simulink model "ventilator"  (R2020a)
settings: Solver=VariableStepAuto  StartTime=0.0  StopTime=20  FixedStep=0.001  MaxStep=0.01  RelTol=1e-3  AbsTol=1e-3
PreLoadFcn:
  | addpath('../controller');
PostLoadFcn:
  | load('params');
InitFcn:
  | load('params');
  | 
  | Transport_Delay = 0.001; % s
  | 
  | P_supply = 4; % bar
  | P_regulator = 0.75; % bar
  | FiO2 = 0.6;
  | 
  | Sensors_Ts = 0.01; % s
  | Zephyr_FS = 50; % SLPM
  | HSC_LP_FS = 160; % mbar
  | HSC_HP_FS = 10000; % mbar
  | 
  | HEPA_ratio = 5 / 20; % mbar / L/min
  | 
  | T_room = 20; % degC
  | RH_room = 0.1;
  | T_humidifier = 40; % degC
  | T_body = 37; % degC
  | 
  | L_tube = 1; % m
  | D_tube = 0.022; % m
  | L_trachea = 0.15; % m
  | D_trachea = 0.015; % m
  | 
  | Chamber_volume = 0.2; % L
  | FRC = 2; % L
  | 
  | cmH2O_to_Pa = 98.0665;
undefined symbols (not defined in the file or in its folder): tc, zephyr
libraries: fl_lib x158, nesl_utility x18, simulink x2
(part 1 of 3)
CloseFcn:
  | clear Transport_Delay
  | clear P_supply P_regulator FiO2
  | clear Sensors_Ts Zephyr_FS HSC_LP_FS HSC_HP_FS
  | clear HEPA_ratio
  | clear T_room RH_room T_humidifier T_body
  | clear L_tube D_tube L_trachea D_trachea
  | clear Chamber_volume FRC
  | clear cmH2O_to_Pa
  | 
  | rmpath('../controller');
Description:
  | Medical Ventilator IIT-Ferrari-Camozzi
settings Model: Creator=MathWorks  LastModifiedBy=upattacini
settings SolverCC: AutoScaleAbsTol=off  MaxConsecutiveMinStep=10  ZeroCrossAlgorithm=Adaptive  AlgebraicLoopSolver=LineSearch
settings DataIOCC: SaveOutput=off  SignalLogging=off  DSMLogging=off  SaveTime=off  ReturnWorkspaceOutputs=off
settings DebuggingCC: IgnoredZcDiagnostic=none  PregeneratedLibrarySubsystemCodeDiagnostic=none  ArithmeticOperatorsInVariantConditions=warning
settings SFSimCC: SimUseLocalCustomCode=off  CustomCodeUndefinedFunction=UseInterfaceOnly
settings RTWCC: RTWUseLocalCustomCode=off
settings SimscapeCC: SimscapeLogName=simlog_ventilator  SimscapeLogDataHistory=10000

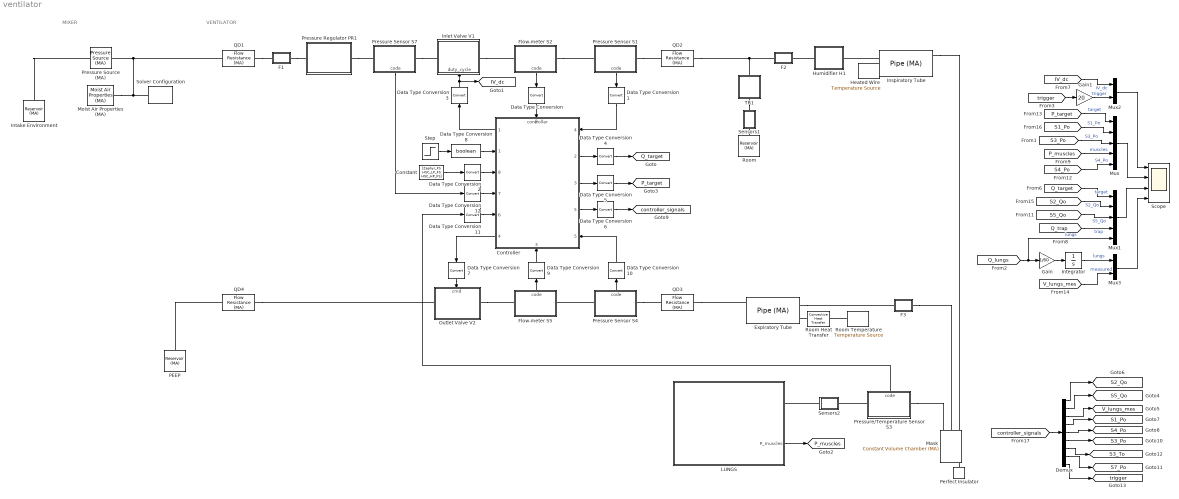
== system ventilator ==
  note: MIXER
  note: VENTILATOR
  Constant : Constant  Value=[Zephyr_FS HSC_LP_FS HSC_HP_FS]
  Controller : ModelReference  ModelNameDialog=controller.slx  SimulationMode=Normal  ModelReferenceVersion=1.393
      settings: PortSchema="{\"entries\":[{\"content\":{\"sides\":[{\"content\":{\"connectorIds\":[\"Out1\",\"In1\",\"In8\",\"In7\",\"In6\",\"Out4\"]},\"type\":\"ConnectorPlacement.EquallySpacedRectSide\",\"uuid\":\"dfd9e8e3-11ff-4499-8101-aea092fe61dc\"},{\"content\":{\"connectorIds\":[\"In4\",\"Out2\",\"Out3\",\"Out5\",\"In5\"],\"side\":\"RIGHT\"},\"type\":\"ConnectorPlacement.EquallySpacedRectSide\",\"uuid\":\"77ce251b-d568-4b78-9724-05f123a60627\"},{\"content\":{\"connectorIds\":[\"In2\"],\"side\":\"TOP\"},\"type\":\"ConnectorPlacement.EquallySpacedRectSide\",\"uuid\":\"86366d86-38ff-4f13-9006-68bedaa415c8\"},{\"content\":{\"connectorIds\":[\"In3\"],\"side\":\"BOTTOM\"},\"type\":\"ConnectorPlacement.EquallySpacedRectSide\",\"uuid\":\"bf42dafa-2a5f-47c5-a086-0e16cdc85087\"}]},\"type\":\"ConnectorPlacement.EquallySpacedConnector\",\"uuid\":\"7cf5e0c6-4e76-497f-b162-c8492159840b\"}],\"packageUris\":[\"http://schema.mathworks.com/mf0/Connector/19700101\"],\"version\":\"1.0\"}"
  Data Type Conversion{,1..7,9..12} (12 alike) : DataTypeConversion
  Data Type Conversion8 : DataTypeConversion  OutDataTypeStr=boolean
  Demux : Demux  Outputs=9
  Expiratory Tube : fl_lib/Moist Air/Elements/Pipe (MA)  length=L_tube m  area=pi*D_tube^2/4 m^2  Dh=D_tube m  length_add=0.1 m  roughness=15e-6 m  Re_lam=2000  Re_tur=4000  shape_factor=64  Nu_lam=3.66  RH_ws=1  time_constant=1e-3 s  moisture_trace_gas_source=foundation.enum.moisture_trace_gas_source.none  moisture_source_spec=foundation.enum.moisture_source_spec.vapor  moisture_mass_flow=0 kg/s  moisture_temperature_spec=foundation.enum.temperature_spec.atmospheric  moisture_temperature=293.15 K  trace_gas_mass_flow=0 kg/s  trace_gas_temperature_spec=foundation.enum.temperature_spec.atmospheric  trace_gas_temperature=293.15 K  p_I_specify=off  p_I_priority=High  p_I=0.101325 MPa  p_I_nominal_specify=off  p_I_nominal_unit=MPa  p_I_nominal_value=1  T_I_specify=on  T_I_priority=High  T_I=T_room degC  T_I_nominal_specify=off  T_I_nominal_unit=K  T_I_nominal_value=1  RH_I_specify=on  RH_I_priority=High  RH_I=RH_room  RH_I_nominal_specify=off  RH_I_nominal_unit=1  RH_I_nominal_value=1  x_w_I_specify=off  x_w_I_priority=None  x_w_I=0  x_w_I_nominal_specify=off  x_w_I_nominal_unit=1  x_w_I_nominal_value=1  y_w_I_specify=off  y_w_I_priority=None  y_w_I=0  y_w_I_nominal_specify=off  y_w_I_nominal_unit=1  y_w_I_nominal_value=1  HR_I_specify=off  HR_I_priority=None  HR_I=0  HR_I_nominal_specify=off  HR_I_nominal_unit=1  HR_I_nominal_value=1  x_g_I_specify=off  x_g_I_priority=High  x_g_I=0  x_g_I_nominal_specify=off  x_g_I_nominal_unit=1  x_g_I_nominal_value=1  y_g_I_specify=off  y_g_I_priority=None  y_g_I=0  y_g_I_nominal_specify=off  y_g_I_nominal_unit=1  y_g_I_nominal_value=1
      settings: SourceProductBaseCode=MT,SS
  F1 : Subsystem  mask(Filter){ratio=HEPA_ratio}
      mask prompts: ratio "Pressure Loss / Fow Ratio (mbar / L/m)"
      mask help: HEPA air filtering.
  F2 : Subsystem  mask(Filter){ratio=HEPA_ratio}
      mask prompts: ratio "Pressure Loss / Fow Ratio (mbar / L/m)"
      mask help: HEPA air filtering.
  F3 : Subsystem  mask(Filter){ratio=HEPA_ratio}
      mask prompts: ratio "Pressure Loss / Fow Ratio (mbar / L/m)"
      mask help: HEPA air filtering.
  Flow-meter S2 : Subsystem  mask(Zephyr Airflow){FS=Zephyr_FS, Ts=Sensors_Ts}
      mask prompts: FS "Full Scale (SLPM)"; Ts "Sample Time (s)"
      mask help: Flow-meter with given characteristics.
      settings: PortSchema="{\"entries\":[{\"content\":{\"sides\":[{\"content\":{\"connectorIds\":[\"LConn1\"]},\"type\":\"ConnectorPlacement.EquallySpacedRectSide\",\"uuid\":\"3eddd698-891c-467d-aa25-3b16d36954ee\"},{\"content\":{\"connectorIds\":[\"RConn1\"],\"side\":\"RIGHT\"},\"type\":\"ConnectorPlacement.EquallySpacedRectSide\",\"uuid\":\"03609a73-c50b-4e66-9a76-94e8c0ebe662\"},{\"content\":{\"connectorIds\":[],\"side\":\"TOP\"},\"type\":\"ConnectorPlacement.EquallySpacedRectSide\",\"uuid\":\"5e48618e-d044-446b-90d3-a440c85d800d\"},{\"content\":{\"connectorIds\":[\"Out1\"],\"side\":\"BOTTOM\"},\"type\":\"ConnectorPlacement.EquallySpacedRectSide\",\"uuid\":\"0cc54025-99cb-4d46-b4e7-784a240d207c\"}]},\"type\":\"ConnectorPlacement.EquallySpacedConnector\",\"uuid\":\"f0fac613-21b7-4ef5-8119-2acb00be7d29\"}],\"packageUris\":[\"http://schema.mathworks.com/mf0/Connector/19700101\"],\"version\":\"1.0\"}"
      mask Display: image('../assets/honeywell.png');
  Flow-meter S5 : Subsystem  mask(Zephyr Airflow){FS=Zephyr_FS, Ts=Sensors_Ts}
      mask prompts: FS "Full Scale (SLPM)"; Ts "Sample Time (s)"
      mask help: Flow-meter with given characteristics.
      settings: PortSchema="{\"entries\":[{\"content\":{\"sides\":[{\"content\":{\"connectorIds\":[\"LConn1\"]},\"type\":\"ConnectorPlacement.EquallySpacedRectSide\",\"uuid\":\"3eddd698-891c-467d-aa25-3b16d36954ee\"},{\"content\":{\"connectorIds\":[\"RConn1\"],\"side\":\"RIGHT\"},\"type\":\"ConnectorPlacement.EquallySpacedRectSide\",\"uuid\":\"03609a73-c50b-4e66-9a76-94e8c0ebe662\"},{\"content\":{\"connectorIds\":[],\"side\":\"TOP\"},\"type\":\"ConnectorPlacement.EquallySpacedRectSide\",\"uuid\":\"5e48618e-d044-446b-90d3-a440c85d800d\"},{\"content\":{\"connectorIds\":[\"Out1\"],\"side\":\"BOTTOM\"},\"type\":\"ConnectorPlacement.EquallySpacedRectSide\",\"uuid\":\"0cc54025-99cb-4d46-b4e7-784a240d207c\"}]},\"type\":\"ConnectorPlacement.EquallySpacedConnector\",\"uuid\":\"f0fac613-21b7-4ef5-8119-2acb00be7d29\"}],\"packageUris\":[\"http://schema.mathworks.com/mf0/Connector/19700101\"],\"version\":\"1.0\"}"
      mask Display: image('../assets/honeywell.png');
  Gain : Gain  Gain=1/60
  Gain1 : Gain  Gain=20
  Heated Wire : fl_lib/Thermal/Thermal Sources/Temperature Source  temperature=T_body degC
      settings: SourceProductBaseCode=MT,SS
  Humidifier H1 : Subsystem  Tag=PublishSubsystem  mask(Humidifier){T_water=T_humidifier, A_humidifier=0.025, V_humidifier=0.001}
      mask prompts: T_water "Water temperature (degC)"; A_humidifier "Water surface area (m^2)"; V_humidifier "Air volume (m^3)"
      mask help: This subsystem models an active passover humidifier to increase moisture in the inspiratory flow.
  Inlet Valve V1 : Subsystem  mask(Proportional Valve){valve_type=CP, ap_tau_em=0.01/4, ap_tau_flow=0.045/4, cp_tau=0.02/4, cp_dead_time=0.01}
      mask prompts: valve_type "Valve Type"; ap_tau_em "Electromechanical Time Constant (s)"; ap_tau_flow "Flow Rate Time Constant (s)"; cp_tau "Time Constant (s)"; cp_dead_time "Dead Time (s)"
      mask help:
      | The valve is characterized by diagrams relating duty cycle, flow rate, and pressure loss.
      | The input is the PWM duty cycle.
      mask init:
      | if valve_type == 1
      |     valve = evalin('base','ap');
      | else
      |     valve = evalin('base','cp');
      | end
      settings: PortSchema="{\"entries\":[{\"content\":{\"sides\":[{\"content\":{\"connectorIds\":[\"LConn1\"]},\"type\":\"ConnectorPlacement.EquallySpacedRectSide\",\"uuid\":\"0b0135b1-d7b1-428e-90f3-2a98bec52953\"},{\"content\":{\"connectorIds\":[\"RConn1\"],\"side\":\"RIGHT\"},\"type\":\"ConnectorPlacement.EquallySpacedRectSide\",\"uuid\":\"8225685a-6f4e-4f4e-a754-9e90146eeb84\"},{\"content\":{\"connectorIds\":[\"In1\"],\"side\":\"TOP\"},\"type\":\"ConnectorPlacement.EquallySpacedRectSide\",\"uuid\":\"19c5f21c-927f-4e6e-aef1-94ad3534e6af\"}]},\"type\":\"ConnectorPlacement.EquallySpacedConnector\",\"uuid\":\"ea880819-6bb4-4c70-964b-d5a8d420d61d\"}],\"packageUris\":[\"http://schema.mathworks.com/mf0/Connector/19700101\"],\"version\":\"1.0\"}"
      mask TypeOptions valve_type: AP | CP
      mask Callback valve_type:
      | numparams = Simulink.Mask.get(gcb).numParameters;
      | enable = cell(1, numparams);
      | enable(:) = {'on'};
      | 
      | mode = get_param(gcb, 'valve_type');
      | if strcmpi(mode, 'CP')
      |     enable(2:3) = {'off'};
      | else
      |     enable(4:5) = {'off'};
      | end
      | set_param(gcb, 'MaskEnables', enable);
      mask Display: image('../assets/camozzi.jpg');
  Inspiratory Tube : fl_lib/Moist Air/Elements/Pipe (MA)  length=L_tube m  area=pi*D_tube^2/4 m^2  Dh=D_tube m  length_add=0.1 m  roughness=15e-6 m  Re_lam=2000  Re_tur=4000  shape_factor=64  Nu_lam=3.66  RH_ws=1  time_constant=1e-3 s  moisture_trace_gas_source=foundation.enum.moisture_trace_gas_source.none  moisture_source_spec=foundation.enum.moisture_source_spec.vapor  moisture_mass_flow=0 kg/s  moisture_temperature_spec=foundation.enum.temperature_spec.atmospheric  moisture_temperature=293.15 K  trace_gas_mass_flow=0 kg/s  trace_gas_temperature_spec=foundation.enum.temperature_spec.atmospheric  trace_gas_temperature=293.15 K  p_I_specify=off  p_I_priority=High  p_I=0.101325 MPa  p_I_nominal_specify=off  p_I_nominal_unit=MPa  p_I_nominal_value=1  T_I_specify=on  T_I_priority=High  T_I=T_room degC  T_I_nominal_specify=off  T_I_nominal_unit=K  T_I_nominal_value=1  RH_I_specify=on  RH_I_priority=High  RH_I=RH_room  RH_I_nominal_specify=off  RH_I_nominal_unit=1  RH_I_nominal_value=1  x_w_I_specify=off  x_w_I_priority=None  x_w_I=0  x_w_I_nominal_specify=off  x_w_I_nominal_unit=1  x_w_I_nominal_value=1  y_w_I_specify=off  y_w_I_priority=None  y_w_I=0  y_w_I_nominal_specify=off  y_w_I_nominal_unit=1  y_w_I_nominal_value=1  HR_I_specify=off  HR_I_priority=None  HR_I=0  HR_I_nominal_specify=off  HR_I_nominal_unit=1  HR_I_nominal_value=1  x_g_I_specify=off  x_g_I_priority=High  x_g_I=0  x_g_I_nominal_specify=off  x_g_I_nominal_unit=1  x_g_I_nominal_value=1  y_g_I_specify=off  y_g_I_priority=None  y_g_I=0  y_g_I_nominal_specify=off  y_g_I_nominal_unit=1  y_g_I_nominal_value=1
      settings: SourceProductBaseCode=MT,SS
  Intake Environment : fl_lib/Moist Air/Elements/Reservoir (MA)  pressure_spec=foundation.enum.pressure_spec.atmospheric  reservoir_pressure=P_supply bar  temperature_spec=foundation.enum.temperature_spec.specified  reservoir_temperature=T_room degC  moisture_spec=foundation.enum.moisture_spec.relative_humidity  reservoir_RH=RH_room  reservoir_x_w=0.01  reservoir_y_w=0.01  reservoir_HR=0.01  trace_gas_spec=foundation.enum.trace_gas_spec.mole_fraction  reservoir_x_g=0  reservoir_y_g=FiO2  RH_ws=1  area_A=pi*D_tube^2/4 m^2
      settings: SourceProductBaseCode=MT,SS
  Integrator : Integrator
  LUNGS : Subsystem  mask(Lungs){lungs_type=Medium, muscles_enabled=off, p_muscles_mag=10, t_inhale=0.5, t_exhale=1, period=5, delay=1.1}
      mask prompts: lungs_type "Lungs Type"; muscles_enabled "Enable Muscles Pressure"; p_muscles_mag "Muscles pressure magnitude (cmH20)"; t_inhale "Inhalation duration (s)"; t_exhale "Exhalation duration (s)"; period "Period (s)"; delay "Delay (s)"
      mask help:
      | This subsystem accounts for the lungs dynamics resorting to a translational mechanical converter that is responsible for converting moist air in volume change.
      |
      | Because the interface cross-sectional area parameter is set to 1 m^2, therefore 1 m of measured displacement is equivalent to 1 m^3 of lungs volume and 1 N of measured force is equivalent to 1 Pa of pressure.
      mask init:
      | lungs_compliant = struct('Em',60,'E',2.6,'Rm',0.9,'R0',0.47,'Kv',-0.45,'Kf',0.01);
      | lungs_medium = struct('Em',60,'E',5.9,'Rm',0.4,'R0',0.3,'Kv',-0.35,'Kf',0.4);
      | lungs_stiff = struct('Em',60,'E',9.1,'Rm',0.85,'R0',0.1,'Kv',-0.6,'Kf',0.8);
      | 
      | if lungs_type == 1
      |     lungs = lungs_compliant;
      | elseif lungs_type == 2
      |     lungs = lungs_medium;
      | else
      |     lungs = lungs_stiff;
      | end
      settings: PortSchema="{\"entries\":[{\"content\":{\"sides\":[{\"content\":{\"connectorIds\":[]},\"type\":\"ConnectorPlacement.EquallySpacedRectSide\",\"uuid\":\"d76c9f72-7b8e-4684-b79a-2f479b0f4ef9\"},{\"content\":{\"connectorIds\":[\"RConn1\",\"Out1\"],\"side\":\"RIGHT\"},\"type\":\"ConnectorPlacement.EquallySpacedRectSide\",\"uuid\":\"9c49ecd1-09fc-45b8-94ed-4278a65fc871\"},{\"content\":{\"connectorIds\":[],\"side\":\"TOP\"},\"type\":\"ConnectorPlacement.EquallySpacedRectSide\",\"uuid\":\"c20a617e-bdd3-44e9-88c4-f17e0ef57963\"}]},\"type\":\"ConnectorPlacement.EquallySpacedConnector\",\"uuid\":\"46ba8907-2938-4721-a0f5-c6c7a7a60368\"}],\"packageUris\":[\"http://schema.mathworks.com/mf0/Connector/19700101\"],\"version\":\"1.0\"}"
      mask TypeOptions lungs_type: Compliant | Medium | Stiff
      mask Callback muscles_enabled:
      | numparams = Simulink.Mask.get(gcb).numParameters;
      | enable = cell(1, numparams);
      | enable(:) = {'on'};
      | h = Simulink.findBlocks(gcb, 'Name' , 'Muscles Pressure Waveform');
      | 
      | mode = get_param(gcb, 'muscles_enabled');
      | if strcmpi(mode, 'on')
      |     set_param(h, 'Commented', 'off');
      | else
      |     set_param(h, 'Commented', 'on');
      |     enable(3:end) = {'off'};
      | end
      | set_param(gcb, 'MaskEnables', enable);
      mask DialogControl Container1 Prompt: Parameters
      mask Display: image('../assets/lungs.png');
  Mask : fl_lib/Moist Air/Elements/Constant Volume Chamber (MA)  volume=Chamber_volume l  num_ports=foundation.enum.num_ports.three  area_A=pi*D_trachea^2/4 m^2  area_B=pi*D_tube^2/4 m^2  area_C=pi*D_tube^2/4 m^2  area_D=0.01 m^2  RH_ws=1  time_constant=1e-3 s  moisture_trace_gas_source=foundation.enum.moisture_trace_gas_source.none  moisture_source_spec=foundation.enum.moisture_source_spec.vapor  moisture_mass_flow=0 kg/s  moisture_temperature_spec=foundation.enum.temperature_spec.atmospheric  moisture_temperature=293.15 K  trace_gas_mass_flow=0 kg/s  trace_gas_temperature_spec=foundation.enum.temperature_spec.atmospheric  trace_gas_temperature=293.15 K  p_I_specify=off  p_I_priority=High  p_I=0.101325 MPa  p_I_nominal_specify=off  p_I_nominal_unit=MPa  p_I_nominal_value=1  T_I_specify=on  T_I_priority=High  T_I=T_room degC  T_I_nominal_specify=off  T_I_nominal_unit=K  T_I_nominal_value=1  RH_I_specify=on  RH_I_priority=High  RH_I=RH_room  RH_I_nominal_specify=off  RH_I_nominal_unit=1  RH_I_nominal_value=1  x_w_I_specify=off  x_w_I_priority=None  x_w_I=0  x_w_I_nominal_specify=off  x_w_I_nominal_unit=1  x_w_I_nominal_value=1  y_w_I_specify=off  y_w_I_priority=None  y_w_I=0  y_w_I_nominal_specify=off  y_w_I_nominal_unit=1  y_w_I_nominal_value=1  HR_I_specify=off  HR_I_priority=None  HR_I=0  HR_I_nominal_specify=off  HR_I_nominal_unit=1  HR_I_nominal_value=1  x_g_I_specify=off  x_g_I_priority=High  x_g_I=0  x_g_I_nominal_specify=off  x_g_I_nominal_unit=1  x_g_I_nominal_value=1  y_g_I_specify=off  y_g_I_priority=None  y_g_I=0  y_g_I_nominal_specify=off  y_g_I_nominal_unit=1  y_g_I_nominal_value=1
      settings: SourceProductBaseCode=MT,SS  InternalSimscapePortConfiguration="{\"Bottom\":[],\"Left\":[{\"id\":\"A\",\"label\":\"A\",\"type\":\"foundation.moist_air.moist_air\"},{\"id\":\"B\",\"label\":\"B\",\"type\":\"foundation.moist_air.moist_air\"},{\"id\":\"C\",\"label\":\"C\",\"type\":\"foundation.moist_air.moist_air\"}],\"Right\":[{\"id\":\"W\",\"label\":\"W\",\"type\":\"output\"},{\"id\":\"F\",\"label\":\"F\",\"type\":\"output\"},{\"id\":\"H\",\"label\":\"H\",\"type\":\"foundation.thermal.thermal\"}],\"Top\":[]}"
  Moist Air Properties (MA) : fl_lib/Moist Air/Utilities/Moist Air Properties (MA)  trace_gas_model=foundation.enum.trace_gas_model.track_properties  R_a=287.047 J/kg/K  R_w=461.523 J/kg/K  R_g=O2.R J/kg/K  T_TLU=[-56.55, -50 : 10 : -10, -5 : 1 : 5, 10 : 10 : 350]' degC  p_ws_TLU=[1.71168953425982e-06; 3.93770601979424e-06; 1.28411717710344e-05; 3.80051394873809e-05; .00010323902900209; .000259873810798063; .000401741022116384; .000437454836117844; .000476040820618202; .000517704666185737; .000562664883741207; .000611212677444345; .000657088049117899; .000705987905898279; .000758082381149132; .000813549384183233; .000872574861129522; .00122818386934022; .0023392147667769; .00424668834054807; .00738442748706953; .0123512704340234; .0199458019246787; .0312006356960619; .0474147199263783; .0701823607447713; .10141797792131; .143375967241115; .198665399739302; .270259606559999; .361500961984849; .476101381081492; .618139196722055; .792053183687694; 1.0026345688121; 1.25501792086105; 1.55467186826983; 1.90739066433297; 2.31928772772542; 2.79679245576864; 3.34665187151016; 3.97593907083533; 4.69207105435535; 5.5028394740883; 6.41645928168037; 7.4416425436169; 8.58770832955728; 9.86474556030261; 11.2838558865497; 12.8575218898034; 14.6001810568052; 16.5291642526045] MPa  h_w_vap_TLU=[2836.88241275372; 2837.81392500514; 2838.63937175807; 2838.7309929628; 2838.06905313927; 2836.62597341095; 2835.60023952573; 2835.37006381376; 2835.13143158077; 2834.88429145066; 2834.62859062897; 2500.93420564316; 2498.55329907119; 2496.17495082036; 2493.79885912205; 2491.42474723191; 2489.05236104642; 2477.20875029194; 2453.54955988604; 2429.83856603313; 2406.00136954922; 2381.97406342174; 2357.69101156389; 2333.08088387814; 2308.06565480412; 2282.56034405021; 2256.47287422313; 2229.70428017508; 2202.14968030993; 2173.69998896199; 2144.24368406447; 2113.66758247452; 2081.85585110571; 2048.68725710494; 2014.03141249899; 1977.7449923284; 1939.66849592886; 1899.62342931686; 1857.40930169838; 1812.79975416601; 1765.53721731251; 1715.32525772152; 1661.81700477787; 1604.59703745016; 1543.1534616334; 1476.83692476464; 1404.80240352424; 1325.92091736114; 1238.61667822208; 1140.5102987018; 1027.62017777647; 892.733785613825] kJ/kg  h_a_TLU=[342.416126230579; 349.005511058471; 359.063577249119; 369.119948684177; 379.175469465129; 389.230944678417; 394.258910928084; 395.264534937366; 396.27017101329; 397.275819932805; 398.281482472874; 399.287159410541; 400.292851523015; 401.298559587728; 402.304284382408; 403.310026685143; 404.315787274435; 409.34489180313; 419.404921755863; 429.468036401264; 439.535033154839; 449.606720928652; 459.683919949603; 469.767460521911; 479.858181001348; 489.956925196484; 500.064539372946; 510.181869006204; 520.309755403634; 530.449032296018; 540.60052248087; 550.765034584465; 560.943359995745; 571.136270013102; 581.344513234296; 591.568813210327; 601.809866375885; 612.068340261954; 622.344871990218; 632.640067043998; 642.95449830646; 653.288705353699; 663.643193987949; 674.018435994423; 684.414869104228; 694.832897145098; 705.272890361557; 715.735185886199; 726.220088344236; 736.727870574087; 747.258774447567; 757.813011774199] kJ/kg  h_w_TLU=[2396.55944251649; 2408.68643343608; 2427.1988031141; 2445.702165897; 2464.18429108356; 2482.62529466839; 2491.82135326629; 2493.6580151792; 2495.49372578218; 2497.32843835745; 2499.16210446923; 2500.99462758899; 2502.83092214066; 2504.6665223621; 2506.50140563013; 2508.335548891; 2510.16892865793; 2519.32352241995; 2537.56068088674; 2555.67742615292; 2573.6403223998; 2591.4109179101; 2608.9455037701; 2626.19492016262; 2643.10444358428; 2659.61377634497; 2675.58278696023; 2696.1846256545; 2716.49989553741; 2736.6235210957; 2756.61216047011; 2776.50561773853; 2796.33378922508; 2816.11979583049; 2835.88181423877; 2855.63430574511; 2875.38889327595; 2895.15500577172; 2914.94035964689; 2934.75132290228; 2954.59319330244; 2974.47041285505; 2994.38673458964; 3014.34535328009; 3034.34900867103; 3054.40006755764; 3074.50058946898; 3094.65237953784; 3114.85703128106; 3135.11596137801; 3155.43043805905; 3175.80160435813] kJ/kg  h_g_TLU=O2.h kJ/kg  mu_a_TLU=[14.2568883320012; 14.6140127728333; 15.1517277055779; 15.6806860159119; 16.2012351072083; 16.7137043125028; 16.9670071730589; 17.017438062815; 17.0677930842452; 17.1180725309876; 17.1682766951315; 17.2184058672268; 17.2684603362935; 17.3184403898301; 17.3683463138234; 17.4181783927569; 17.4679369096204; 17.7156358640698; 18.2056751785154; 18.68879035749; 19.1652344664982; 19.6352478927873; 20.099059103658; 20.5568853601578; 21.0089333871663; 21.4554000014051; 21.8964726992323; 22.3323302062775; 22.7631429910631; 23.1890737447833; 23.6102778293792; 24.0269036959922; 24.4390932757886; 24.8469823450548; 25.2507008663546; 25.6503733074314; 26.0461189394339; 26.4380521159325; 26.8262825340948; 27.2109154792923; 27.5920520543128; 27.969789394274; 28.3442208682439; 28.7154362685068; 29.0835219883356; 29.4485611890712; 29.8106339572472; 30.1698174524429; 30.5261860464955; 30.8798114546565; 31.2307628592324; 31.5791070262086] s*uPa  mu_w_TLU=[6.81365662228272; 7.04953750742707; 7.40970098298307; 7.76991278093907; 8.13017290129507; 8.49048134405107; 8.67065368632907; 8.70668960445667; 8.74272600580827; 8.77876289038387; 8.81480025818347; 8.85083810920707; 8.88687644345467; 8.92291526092627; 8.95895456162187; 8.99499434554147; 9.03103461268507; 9.21124319676307; 9.57169660671907; 9.93219833907507; 10.2927483938311; 10.6533467709871; 11.0139934705431; 11.3746884924991; 11.7354318368551; 12.0962235036111; 12.4570634927671; 12.8179518043231; 13.1788884382791; 13.5398733946351; 13.9009066733911; 14.2619882745471; 14.6231181981031; 14.9842964440591; 15.3455230124151; 15.7067979031711; 16.0681211163271; 16.4294926518831; 16.7909125098391; 17.1523806901951; 17.5138971929511; 17.8754620181071; 18.2370751656631; 18.5987366356191; 18.9604464279751; 19.3222045427311; 19.6840109798871; 20.0458657394431; 20.4077688213991; 20.7697202257551; 21.1317199525111; 21.4937680016671] s*uPa  mu_g_TLU=O2.mu s*uPa  k_a_TLU=[19.8808489374933; 20.4162454629695; 21.2248743590758; 22.0232452890903; 22.8117314495857; 23.5906913619588; 23.9767075412237; 24.053639990175; 24.1304826682191; 24.2072359051629; 24.2839000294007; 24.3604753679152; 24.4369622462801; 24.5133609886625; 24.5896719178249; 24.6658953551279; 24.7420316205333; 25.1214164701832; 25.8738283029331; 26.6180150229276; 27.3542674377332; 28.0828634735341; 28.8040686837224; 29.5181367785657; 30.2253101618423; 30.9258204644224; 31.6198890677835; 32.3077276126633; 32.9895384896798; 33.6655153099498; 34.33584335461; 35.0007000027879; 35.6602551380254; 36.3146715334901; 36.9641052165342; 37.6087058133173; 38.248616874307; 38.8839761815308; 39.5149160384798; 40.1415635435708; 40.7640408480637; 41.3824653993118; 41.9969501701893; 42.6076038755117; 43.2145311762238; 43.8178328720941; 44.4176060836121; 45.013944423749; 45.6069381602018; 46.1966743687041; 46.783237077953; 47.3667074066625] mW/m/K  k_w_TLU=[11.46288215976; 11.941997488935; 12.676358586935; 13.414208884935; 14.155548382935; 14.900377080935; 15.274099879935; 15.348949115735; 15.423833243535; 15.498752263335; 15.573706175135; 15.648694978935; 15.723718674735; 15.798777262535; 15.873870742335; 15.948999114135; 16.024162377935; 16.400502076935; 17.155798374935; 17.914583872935; 18.676858570935; 19.442622468935; 20.211875566935; 20.984617864935; 21.760849362935; 22.540570060935; 23.323779958935; 24.110479056935; 24.900667354935; 25.694344852935; 26.491511550935; 27.292167448935; 28.096312546935; 28.903946844935; 29.715070342935; 30.529683040935; 31.347784938935; 32.169376036935; 32.994456334935; 33.823025832935; 34.655084530935; 35.490632428935; 36.329669526935; 37.172195824935; 38.018211322935; 38.867716020935; 39.720709918935; 40.577193016935; 41.437165314935; 42.300626812935; 43.167577510935; 44.038017408935] mW/m/K  k_g_TLU=O2.k mW/m/K  D_w=25 mm^2/s  D_g=O2.d mm^2/s  p_min=1 kPa  p_max=inf MPa  T_min=-56.55 degC  T_max=350 degC  p_atm=0.101325 MPa  T_atm=T_room degC
      settings: SourceProductBaseCode=MT,SS
  Mux : Mux  Inputs=5
  Mux1 : Mux  Inputs=5
  Mux2 : Mux  Inputs=2
  Mux3 : Mux  Inputs=2
  Outlet Valve V2 : Subsystem  mask(CFB ON/OFF Valve){Kv=1, tau=0.02/4}
      mask prompts: Kv "Kv (m^3/h)"; tau "Valve Time Constant (s)"
      mask help:
      | The valve is characterized by the coefficient Kv.
      | The input is the ON/OFF switch.
      settings: PortSchema="{\"entries\":[{\"content\":{\"sides\":[{\"content\":{\"connectorIds\":[\"LConn1\"]},\"type\":\"ConnectorPlacement.EquallySpacedRectSide\",\"uuid\":\"0b0135b1-d7b1-428e-90f3-2a98bec52953\"},{\"content\":{\"connectorIds\":[\"RConn1\"],\"side\":\"RIGHT\"},\"type\":\"ConnectorPlacement.EquallySpacedRectSide\",\"uuid\":\"8225685a-6f4e-4f4e-a754-9e90146eeb84\"},{\"content\":{\"connectorIds\":[\"In1\"],\"side\":\"TOP\"},\"type\":\"ConnectorPlacement.EquallySpacedRectSide\",\"uuid\":\"19c5f21c-927f-4e6e-aef1-94ad3534e6af\"}]},\"type\":\"ConnectorPlacement.EquallySpacedConnector\",\"uuid\":\"ea880819-6bb4-4c70-964b-d5a8d420d61d\"}],\"packageUris\":[\"http://schema.mathworks.com/mf0/Connector/19700101\"],\"version\":\"1.0\"}"
      mask Display: image('../assets/camozzi.jpg');
  PEEP : fl_lib/Moist Air/Elements/Reservoir (MA)  pressure_spec=foundation.enum.pressure_spec.specified  reservoir_pressure=101325 + 5 * cmH2O_to_Pa Pa  temperature_spec=foundation.enum.temperature_spec.specified  reservoir_temperature=T_room degC  moisture_spec=foundation.enum.moisture_spec.relative_humidity  reservoir_RH=RH_room  reservoir_x_w=0.01  reservoir_y_w=0.01  reservoir_HR=0.01  trace_gas_spec=foundation.enum.trace_gas_spec.mass_fraction  reservoir_x_g=0  reservoir_y_g=0.001  RH_ws=1  area_A=pi*D_tube^2/4 m^2
      settings: SourceProductBaseCode=MT,SS
  Perfect Insulator : fl_lib/Thermal/Thermal Elements/Perfect Insulator  T_specify=off  T_priority=None  T=0 K  T_nominal_specify=off  T_nominal_unit=K  T_nominal_value=1
      settings: SourceProductBaseCode=MT,SS
  Pressure Regulator PR1 : Subsystem  mask(Pressure Regulator){Pr=P_regulator}
      mask prompts: Pr "Regulated Pressure (bar)"
      mask help: The regulator is characterized by diagrams relating the inlet pressure, the flow and the regulated pressure.
      mask DialogControl Container1 Prompt: Parameters
      mask Display: image('../assets/camozzi.jpg');
  Pressure Sensor S1 : Subsystem  mask(HSC Sensor){FS=HSC_LP_FS, Ts=Sensors_Ts}
      mask prompts: FS "Full Scale (mbar)"; Ts "Sample Time (s)"
      mask help: Pressure sensor with given characteristics.
      settings: PortSchema="{\"entries\":[{\"content\":{\"sides\":[{\"content\":{\"connectorIds\":[\"LConn1\"]},\"type\":\"ConnectorPlacement.EquallySpacedRectSide\",\"uuid\":\"3eddd698-891c-467d-aa25-3b16d36954ee\"},{\"content\":{\"connectorIds\":[\"RConn1\"],\"side\":\"RIGHT\"},\"type\":\"ConnectorPlacement.EquallySpacedRectSide\",\"uuid\":\"03609a73-c50b-4e66-9a76-94e8c0ebe662\"},{\"content\":{\"connectorIds\":[],\"side\":\"TOP\"},\"type\":\"ConnectorPlacement.EquallySpacedRectSide\",\"uuid\":\"5e48618e-d044-446b-90d3-a440c85d800d\"},{\"content\":{\"connectorIds\":[\"Out1\"],\"side\":\"BOTTOM\"},\"type\":\"ConnectorPlacement.EquallySpacedRectSide\",\"uuid\":\"0cc54025-99cb-4d46-b4e7-784a240d207c\"}]},\"type\":\"ConnectorPlacement.EquallySpacedConnector\",\"uuid\":\"f0fac613-21b7-4ef5-8119-2acb00be7d29\"}],\"packageUris\":[\"http://schema.mathworks.com/mf0/Connector/19700101\"],\"version\":\"1.0\"}"
      mask Display: image('../assets/honeywell.png');
  Pressure Sensor S4 : Subsystem  mask(HSC Sensor){FS=HSC_LP_FS, Ts=Sensors_Ts}
      mask prompts: FS "Full Scale (mbar)"; Ts "Sample Time (s)"
      mask help: Pressure sensor with given characteristics.
      settings: PortSchema="{\"entries\":[{\"content\":{\"sides\":[{\"content\":{\"connectorIds\":[\"LConn1\"]},\"type\":\"ConnectorPlacement.EquallySpacedRectSide\",\"uuid\":\"3eddd698-891c-467d-aa25-3b16d36954ee\"},{\"content\":{\"connectorIds\":[\"RConn1\"],\"side\":\"RIGHT\"},\"type\":\"ConnectorPlacement.EquallySpacedRectSide\",\"uuid\":\"03609a73-c50b-4e66-9a76-94e8c0ebe662\"},{\"content\":{\"connectorIds\":[],\"side\":\"TOP\"},\"type\":\"ConnectorPlacement.EquallySpacedRectSide\",\"uuid\":\"5e48618e-d044-446b-90d3-a440c85d800d\"},{\"content\":{\"connectorIds\":[\"Out1\"],\"side\":\"BOTTOM\"},\"type\":\"ConnectorPlacement.EquallySpacedRectSide\",\"uuid\":\"0cc54025-99cb-4d46-b4e7-784a240d207c\"}]},\"type\":\"ConnectorPlacement.EquallySpacedConnector\",\"uuid\":\"f0fac613-21b7-4ef5-8119-2acb00be7d29\"}],\"packageUris\":[\"http://schema.mathworks.com/mf0/Connector/19700101\"],\"version\":\"1.0\"}"
      mask Display: image('../assets/honeywell.png');
  Pressure Sensor S7 : Subsystem  mask(HSC Sensor){FS=HSC_HP_FS, Ts=Sensors_Ts}
      mask prompts: FS "Full Scale (mbar)"; Ts "Sample Time (s)"
      mask help: Pressure sensor with given characteristics.
      settings: PortSchema="{\"entries\":[{\"content\":{\"sides\":[{\"content\":{\"connectorIds\":[\"LConn1\"]},\"type\":\"ConnectorPlacement.EquallySpacedRectSide\",\"uuid\":\"3eddd698-891c-467d-aa25-3b16d36954ee\"},{\"content\":{\"connectorIds\":[\"RConn1\"],\"side\":\"RIGHT\"},\"type\":\"ConnectorPlacement.EquallySpacedRectSide\",\"uuid\":\"03609a73-c50b-4e66-9a76-94e8c0ebe662\"},{\"content\":{\"connectorIds\":[],\"side\":\"TOP\"},\"type\":\"ConnectorPlacement.EquallySpacedRectSide\",\"uuid\":\"5e48618e-d044-446b-90d3-a440c85d800d\"},{\"content\":{\"connectorIds\":[\"Out1\"],\"side\":\"BOTTOM\"},\"type\":\"ConnectorPlacement.EquallySpacedRectSide\",\"uuid\":\"0cc54025-99cb-4d46-b4e7-784a240d207c\"}]},\"type\":\"ConnectorPlacement.EquallySpacedConnector\",\"uuid\":\"f0fac613-21b7-4ef5-8119-2acb00be7d29\"}],\"packageUris\":[\"http://schema.mathworks.com/mf0/Connector/19700101\"],\"version\":\"1.0\"}"
      mask Display: image('../assets/honeywell.png');
  Pressure Source (MA) : fl_lib/Moist Air/Sources/Pressure Source (MA)  power_spec=foundation.enum.power_spec.none  pressure_differential=P_supply bar  area_A=pi*D_tube^2/4 m^2  area_B=pi*D_tube^2/4 m^2
      settings: SourceProductBaseCode=SS  InternalSimscapePortConfiguration="{\"Bottom\":[],\"Left\":[{\"id\":\"A\",\"label\":\"A\",\"type\":\"foundation.moist_air.moist_air\"}],\"Right\":[{\"id\":\"B\",\"label\":\"B\",\"type\":\"foundation.moist_air.moist_air\"}],\"Top\":[]}"
  Pressure/Temperature Sensor S3 : Subsystem  mask(HSC Sensor){FS=HSC_LP_FS, Ts=Sensors_Ts}
      mask prompts: FS "Pressure Full Scale (mbar)"; Ts "Sample Time (s)"
      mask help: Pressure sensor with given characteristics.
      settings: PortSchema="{\"entries\":[{\"content\":{\"sides\":[{\"content\":{\"connectorIds\":[\"LConn1\"]},\"type\":\"ConnectorPlacement.EquallySpacedRectSide\",\"uuid\":\"3eddd698-891c-467d-aa25-3b16d36954ee\"},{\"content\":{\"connectorIds\":[\"RConn1\"],\"side\":\"RIGHT\"},\"type\":\"ConnectorPlacement.EquallySpacedRectSide\",\"uuid\":\"03609a73-c50b-4e66-9a76-94e8c0ebe662\"},{\"content\":{\"connectorIds\":[],\"side\":\"TOP\"},\"type\":\"ConnectorPlacement.EquallySpacedRectSide\",\"uuid\":\"5e48618e-d044-446b-90d3-a440c85d800d\"},{\"content\":{\"connectorIds\":[\"Out1\"],\"side\":\"BOTTOM\"},\"type\":\"ConnectorPlacement.EquallySpacedRectSide\",\"uuid\":\"0cc54025-99cb-4d46-b4e7-784a240d207c\"}]},\"type\":\"ConnectorPlacement.EquallySpacedConnector\",\"uuid\":\"f0fac613-21b7-4ef5-8119-2acb00be7d29\"}],\"packageUris\":[\"http://schema.mathworks.com/mf0/Connector/19700101\"],\"version\":\"1.0\"}"
      mask Display: image('../assets/honeywell.png');
  QD{1..4} (4 alike) : fl_lib/Moist Air/Elements/Flow Resistance (MA)  delta_p_nominal=20e-3 bar  mdot_nominal=160 * (1.225 * 1e-3/60) kg/s  rho_nominal=1.225 kg/m^3  area=pi*D_tube^2/4 m^2  laminar_fraction=1e-3
      settings: SourceProductBaseCode=MT,SS
  Room : fl_lib/Moist Air/Elements/Reservoir (MA)  pressure_spec=foundation.enum.pressure_spec.atmospheric  reservoir_pressure=0.101325 MPa  temperature_spec=foundation.enum.temperature_spec.specified  reservoir_temperature=T_room degC  moisture_spec=foundation.enum.moisture_spec.relative_humidity  reservoir_RH=RH_room  reservoir_x_w=0.01  reservoir_y_w=0.01  reservoir_HR=0.01  trace_gas_spec=foundation.enum.trace_gas_spec.mass_fraction  reservoir_x_g=0  reservoir_y_g=0.001  RH_ws=1  area_A=pi*D_tube^2/4 m^2
      settings: SourceProductBaseCode=MT,SS
  Room Temperature : fl_lib/Thermal/Thermal Sources/Temperature Source  temperature=T_room degC
      settings: SourceProductBaseCode=MT,SS
  Room Heat Transfer : fl_lib/Thermal/Thermal Elements/Convective Heat Transfer  area=pi*D_tube*L_tube m^2  heat_tr_coeff=20 W/(m^2 * K)  T_specify=off  T_priority=None  T=0 K  T_nominal_specify=off  T_nominal_unit=K  T_nominal_value=1  Q_specify=off  Q_priority=None  Q=0 W  Q_nominal_specify=off  Q_nominal_unit=W  Q_nominal_value=1
      settings: SourceProductBaseCode=MT,SS
  Scope : Scope  NumInputPorts=4
  Sensors1 : Subsystem
  Sensors2 : Subsystem
  Solver Configuration : nesl_utility/Solver Configuration  PhysicalDomain=network_engine_domain  SubClassName=solver  LeftPortType=input  RightPortType=generic  Tones=[]  Harmonics=[]  SimulateNoise=off  Profile=off  UseLocalSampling=off  EnableSwitchedLinearOptims=on  FrequencyDomain=off  UseCCode=off  RelTol=0.001  AbsTol=1e-06  MinStep=1e-09  ToWorkspace=off  RevertToSquareIcSolve=off  NumHomotopyIterations=100  PhasorMode=off  PhasorModeNumHarmonics=1  DoDC=off  ResidualTolerance=1e-9  UseLocalSolver=off  LocalSolverChoice=NE_TRAPEZOIDAL_ADVANCER  LocalSolverSampleTime=0.001  DoFixedCost=off  MaxNonlinIter=3  MaxModeIter=2  LinearAlgebra=auto  EquationFormulation=NE_TIME_EF  DelaysMemoryBudget=1024  AutomaticFiltering=on  FilteringTimeConstant=0.001  PartitionStorageMethod=AS_NEEDED  PartitionMemoryBudget=1024  PartitionMethod=FAST
      settings: SourceProductBaseCode=MT,SS
  Step : Step  Time=0  OutDataTypeStr=single  SampleTime=0
  TR1 : Subsystem  Tag=PublishSubsystem  mask(Check Valve){p_max=80.01 * cmH2O_to_Pa, p_crack=80 * cmH2O_to_Pa, D_nozzle=0.9*D_tube, tau=0.001}
      mask prompts: p_max "Max opening pressure differential (Pa)"; p_crack "Cracking pressure differential (Pa)"; D_nozzle "Nozzle Diameter (m)"; tau "Valve Time Constant (s)"
      mask help: This subsystem models a check valve that permits flow from port A to port B but restricts flow from port B to port A.
      mask Display:
      | plot([215.221090475097;214.952657515928;214.149943794556;212.820679882927;210.97766731916;208.638655321736;205.826169854825;202.567296690933;198.893420560112;194.839922897845;190.445841102487;185.753492583777;180.808067223049;175.657192169971;170.350473167059;164.939016819259;159.474938409403;154.010859999547;148.599403651747;143.292684648835;138.141809595757;133.196384235029;128.504035716319;124.109953920961;120.056456258694;116.382580127872;113.123706963981;110.31122149707;107.972209499646;106.129196935879;104.79993302425;103.997219302878;103.728786343709;103.997219302878;104.79993302425;106.129196935879;107.972209499646;110.31122149707;113.123706963981;116.382580127873;120.056456258694;124.109953920961;128.504035716319;133.196384235029;138.141809595757;143.292684648835;148.599403651747;154.010859999547;159.474938409403;164.939016819259;170.350473167059;175.657192169971;180.808067223049;185.753492583777;190.445841102487;194.839922897845;198.893420560112;202.567296690933;205.826169854824;208.638655321736;210.97766731916;212.820679882927;214.149943794556;214.952657515928;215.221090475097;215.221090475097], [110.78366660513;105.319588195274;99.9081318474735;94.6014128445616;89.4505377914837;84.5051124307557;79.8127639120459;75.418682116688;71.3651844544209;67.6913083235994;64.4324351597082;61.619949692797;59.280937695373;57.4379251316055;56.1086612199767;55.3059474986051;55.0375145394355;55.3059474986051;56.1086612199767;57.4379251316055;59.2809376953731;61.619949692797;64.4324351597083;67.6913083235994;71.365184454421;75.418682116688;79.8127639120459;84.5051124307557;89.4505377914838;94.6014128445617;99.9081318474736;105.319588195274;110.78366660513;116.247745014986;121.659201362786;126.965920365698;132.116795418776;137.062220779504;141.754569298214;146.148651093572;150.202148755839;153.87602488666;157.134898050551;159.947383517463;162.286395514887;164.129408078654;165.458671990283;166.261385711655;166.529818670824;166.261385711655;165.458671990283;164.129408078654;162.286395514887;159.947383517463;157.134898050551;153.87602488666;150.202148755839;146.148651093572;141.754569298214;137.062220779504;132.116795418776;126.965920365698;121.659201362786;116.247745014986;110.78366660513;110.78366660513])
      | plot([176.923169055954;73.9345152396709;179.757719160989], [200.544419931248;111.728516640142;16.298663103953])
      | plot([75.3202952910215;0.236212508752942], [112.736356677487;112.673366675153])
      | plot([217.047800542787;228.386000962928;242.558751488104;256.731502013281;265.235152328387;270.904252538458;276.573352748528], [112.736356677487;155.254608253017;70.2181051019579;155.254608253017;109.901806572452;70.2181051019579;112.736356677487])
      | patch([370.381213724613;0.472425017505941;0.472425017505884;370.381213724613;370.381213724613;370.853638742119;370.853638742119;0;5.6843418860808e-14;370.853638742119;370.381213724613], [225.819158367813;225.819158367813;0.472425017505884;0.472425017505884;225.819158367813;226.291583385319;0;0;226.291583385319;226.291583385319;225.819158367813], [1;1;1])
      | plot([276.573352748528;370.113506214693], [112.736356677487;112.736356677487])
  tag scope: IV_dc=global, P_muscles=global, P_target=global, Q_target=global, S1_Po=global, S2_Qo=global, S3_Po=global, S3_To=global, S4_Po=global, S5_Qo=global, S7_Po=global, V_lungs_mes=global, controller_signals=global, trigger=global
  wires:
  Mux/1 -> Scope/2
  Mux1/1 -> Scope/3
  Controller/1 -> Data Type Conversion3/1
  Controller/2 -> Data Type Conversion4/1
  Controller/4 -> Data Type Conversion7/1
  Controller/3 -> Data Type Conversion5/1
  Controller/5 -> Data Type Conversion6/1
  Demux/1 -> [S2_Qo]
  Flow-meter S2/1(code) -> Data Type Conversion/1
  Data Type Conversion8/1 -> Controller/1
  Pressure Sensor S1/1(code) -> Data Type Conversion1/1
  Data Type Conversion4/1 -> [Q_target]
  Data Type Conversion5/1 -> [P_target]
  Data Type Conversion7/1 -> Outlet Valve V2/1(cmd)
  Step/1 -> Data Type Conversion8/1
  Data Type Conversion1/1 -> Controller/4
  Data Type Conversion/1 -> Controller/2
  Demux/2 -> [S5_Qo]
  Data Type Conversion9/1 -> Controller/3
  Flow-meter S5/1(code) -> Data Type Conversion9/1
  Data Type Conversion10/1 -> Controller/5
  Pressure Sensor S4/1(code) -> Data Type Conversion10/1
  Demux/4 -> [S1_Po]
  Demux/5 -> [S4_Po]
  Demux/3 -> [V_lungs_mes]
  Integrator/1 -> Mux3/1  "lungs"
  [V_lungs_mes] -> Mux3/2  "measured"
  Mux3/1 -> Scope/4
  Constant/1 -> Data Type Conversion2/1
  Data Type Conversion6/1 -> [controller_signals]
  [controller_signals] -> Demux/1
  Data Type Conversion3/1 -> Inlet Valve V1/1(duty_cycle), [IV_dc]
  Data Type Conversion11/1 -> Controller/6
  Pressure/Temperature Sensor S3/1(code) -> Data Type Conversion11/1
  Demux/6 -> [S3_Po]
  [Q_target] -> Mux1/1  "target"
  [S5_Qo] -> Mux1/3  "S5_Qo"
  [S2_Qo] -> Mux1/2  "S2_Qo"
  Data Type Conversion2/1 -> Controller/8
  Data Type Conversion12/1 -> Controller/7
  Pressure Sensor S7/1(code) -> Data Type Conversion12/1
  [S3_Po] -> Mux/3  "S3_Po"
  [P_muscles] -> Mux/4  "muscles"
  [S1_Po] -> Mux/2  "S1_Po"
  [P_target] -> Mux/1  "target"
  [S4_Po] -> Mux/5  "S4_Po"
  Demux/7 -> [S3_To]
  Demux/8 -> [S7_Po]
  [Q_lungs] -> Mux1/5, Gain/1  "lungs"
  Gain/1 -> Integrator/1
  LUNGS/1(P_muscles) -> [P_muscles]
  Demux/9 -> [trigger]
  [Q_trap] -> Mux1/4  "trap"
  Mux2/1 -> Scope/1
  [IV_dc] -> Mux2/1  "IV_dc"
  [trigger] -> Gain1/1
  Gain1/1 -> Mux2/2  "trigger"
  connections:
  Humidifier H1/LConn1 -- F2/RConn1
  Inspiratory Tube/LConn1 -- Humidifier H1/RConn1
  Heated Wire/LConn1 -- Inspiratory Tube/LConn2
  Room Heat Transfer/LConn1 -- Expiratory Tube/LConn2
  Room Temperature/LConn1 -- Room Heat Transfer/RConn1
  Mask/RConn3 -- Perfect Insulator/LConn1
  Expiratory Tube/LConn1 -- F3/RConn1
  Pressure/Temperature Sensor S3/LConn1 -- Mask/LConn1
  TR1/LConn1 -- QD2/RConn1 -- F2/LConn1
  F3/LConn1 -- Mask/LConn2
  Outlet Valve V2/LConn1 -- Flow-meter S5/RConn1
  Room/LConn1 -- Sensors1/RConn1
  QD3/LConn1 -- Expiratory Tube/RConn1
  QD4/RConn1 -- PEEP/LConn1
  TR1/RConn1 -- Sensors1/LConn1
  QD4/LConn1 -- Outlet Valve V2/RConn1
  Pressure Sensor S4/LConn1 -- QD3/RConn1
  Pressure Sensor S4/RConn1 -- Flow-meter S5/LConn1
  Pressure/Temperature Sensor S3/RConn1 -- Sensors2/LConn1
  QD1/RConn1 -- F1/LConn1
  Solver Configuration/RConn1 -- Moist Air Properties (MA)/RConn1 -- Pressure Source (MA)/RConn1 -- QD1/LConn1
  Pressure Source (MA)/LConn1 -- Intake Environment/LConn1
  Inspiratory Tube/RConn1 -- Mask/LConn3
  Pressure Sensor S1/RConn1 -- QD2/LConn1
  Flow-meter S2/RConn1 -- Pressure Sensor S1/LConn1
  Inlet Valve V1/RConn1 -- Flow-meter S2/LConn1
  Sensors2/RConn1 -- LUNGS/RConn1
  F1/RConn1 -- Pressure Regulator PR1/LConn1
  Pressure Regulator PR1/RConn1 -- Pressure Sensor S7/LConn1
  Pressure Sensor S7/RConn1 -- Inlet Valve V1/LConn1

== system ventilator/F1 ==
  Controlled Pressure Source (MA) : fl_lib/Moist Air/Sources/Controlled Pressure Source (MA)  power_spec=foundation.enum.power_spec.none  area_A=pi*D_tube^2/4 m^2  area_B=pi*D_tube^2/4 m^2
      settings: SourceProductBaseCode=SS  InternalSimscapePortConfiguration="{\"Bottom\":[],\"Left\":[{\"id\":\"A\",\"label\":\"A\",\"type\":\"foundation.moist_air.moist_air\"},{\"id\":\"P\",\"label\":\"P\",\"type\":\"input\"}],\"Right\":[{\"id\":\"B\",\"label\":\"B\",\"type\":\"foundation.moist_air.moist_air\"}],\"Top\":[]}"
  PS Gain : fl_lib/Physical Signals/Functions/PS Gain  gain=- 1e3/(1/60) * 100 * ratio Pa/(m^3/s)
  Volumetric Flow Rate Sensor (MA) : fl_lib/Moist Air/Sensors/Volumetric Flow Rate Sensor (MA)  volumetric_flow_conditions=foundation.enum.volumetric_flow_conditions.actual  p_std=0.101325 MPa  T_std=20 degC  RH_std=0.65
      settings: SourceProductBaseCode=MT,SS  InternalSimscapePortConfiguration="{\"Bottom\":[],\"Left\":[{\"id\":\"A\",\"label\":\"A\",\"type\":\"foundation.moist_air.moist_air\"}],\"Right\":[{\"id\":\"B\",\"label\":\"B\",\"type\":\"foundation.moist_air.moist_air\"},{\"id\":\"V\",\"label\":\"V\",\"type\":\"output\"}],\"Top\":[]}"
  A : PMIOPort  Side=Left
  B : PMIOPort  Port=2  Side=Right
  connections:
  PS Gain/RConn1 -- Controlled Pressure Source (MA)/LConn2
  Volumetric Flow Rate Sensor (MA)/RConn2 -- PS Gain/LConn1
  Controlled Pressure Source (MA)/RConn1 -- B/RConn1
  Controlled Pressure Source (MA)/LConn1 -- Volumetric Flow Rate Sensor (MA)/RConn1
  Volumetric Flow Rate Sensor (MA)/LConn1 -- A/RConn1

== system ventilator/F2 ==
  Controlled Pressure Source (MA) : fl_lib/Moist Air/Sources/Controlled Pressure Source (MA)  power_spec=foundation.enum.power_spec.none  area_A=pi*D_tube^2/4 m^2  area_B=pi*D_tube^2/4 m^2
      settings: SourceProductBaseCode=SS  InternalSimscapePortConfiguration="{\"Bottom\":[],\"Left\":[{\"id\":\"A\",\"label\":\"A\",\"type\":\"foundation.moist_air.moist_air\"},{\"id\":\"P\",\"label\":\"P\",\"type\":\"input\"}],\"Right\":[{\"id\":\"B\",\"label\":\"B\",\"type\":\"foundation.moist_air.moist_air\"}],\"Top\":[]}"
  PS Gain : fl_lib/Physical Signals/Functions/PS Gain  gain=- 1e3/(1/60) * 100 * ratio Pa/(m^3/s)
  Volumetric Flow Rate Sensor (MA) : fl_lib/Moist Air/Sensors/Volumetric Flow Rate Sensor (MA)  volumetric_flow_conditions=foundation.enum.volumetric_flow_conditions.actual  p_std=0.101325 MPa  T_std=20 degC  RH_std=0.65
      settings: SourceProductBaseCode=MT,SS  InternalSimscapePortConfiguration="{\"Bottom\":[],\"Left\":[{\"id\":\"A\",\"label\":\"A\",\"type\":\"foundation.moist_air.moist_air\"}],\"Right\":[{\"id\":\"B\",\"label\":\"B\",\"type\":\"foundation.moist_air.moist_air\"},{\"id\":\"V\",\"label\":\"V\",\"type\":\"output\"}],\"Top\":[]}"
  A : PMIOPort  Side=Left
  B : PMIOPort  Port=2  Side=Right
  connections:
  Volumetric Flow Rate Sensor (MA)/LConn1 -- A/RConn1
  Controlled Pressure Source (MA)/LConn1 -- Volumetric Flow Rate Sensor (MA)/RConn1
  Controlled Pressure Source (MA)/RConn1 -- B/RConn1
  Volumetric Flow Rate Sensor (MA)/RConn2 -- PS Gain/LConn1
  PS Gain/RConn1 -- Controlled Pressure Source (MA)/LConn2

== system ventilator/F3 ==
  Controlled Pressure Source (MA) : fl_lib/Moist Air/Sources/Controlled Pressure Source (MA)  power_spec=foundation.enum.power_spec.none  area_A=pi*D_tube^2/4 m^2  area_B=pi*D_tube^2/4 m^2
      settings: SourceProductBaseCode=SS  InternalSimscapePortConfiguration="{\"Bottom\":[],\"Left\":[{\"id\":\"A\",\"label\":\"A\",\"type\":\"foundation.moist_air.moist_air\"},{\"id\":\"P\",\"label\":\"P\",\"type\":\"input\"}],\"Right\":[{\"id\":\"B\",\"label\":\"B\",\"type\":\"foundation.moist_air.moist_air\"}],\"Top\":[]}"
  PS Gain : fl_lib/Physical Signals/Functions/PS Gain  gain=- 1e3/(1/60) * 100 * ratio Pa/(m^3/s)
  Volumetric Flow Rate Sensor (MA) : fl_lib/Moist Air/Sensors/Volumetric Flow Rate Sensor (MA)  volumetric_flow_conditions=foundation.enum.volumetric_flow_conditions.actual  p_std=0.101325 MPa  T_std=20 degC  RH_std=0.65
      settings: SourceProductBaseCode=MT,SS  InternalSimscapePortConfiguration="{\"Bottom\":[],\"Left\":[{\"id\":\"A\",\"label\":\"A\",\"type\":\"foundation.moist_air.moist_air\"}],\"Right\":[{\"id\":\"B\",\"label\":\"B\",\"type\":\"foundation.moist_air.moist_air\"},{\"id\":\"V\",\"label\":\"V\",\"type\":\"output\"}],\"Top\":[]}"
  A : PMIOPort  Side=Left
  B : PMIOPort  Port=2  Side=Right
  connections:
  PS Gain/RConn1 -- Controlled Pressure Source (MA)/LConn2
  Volumetric Flow Rate Sensor (MA)/RConn2 -- PS Gain/LConn1
  Controlled Pressure Source (MA)/RConn1 -- B/RConn1
  Controlled Pressure Source (MA)/LConn1 -- Volumetric Flow Rate Sensor (MA)/RConn1
  Volumetric Flow Rate Sensor (MA)/LConn1 -- A/RConn1
